simulink model "test"  (Simulink 8.4)
settings: Solver=ode45  StartTime=0.0  StopTime=10.0  RelTol=1e-3
settings Model: Creator=fanwenjun  LastModifiedBy=fanwenjun
settings DataIOCC: SignalLoggingSaveFormat=Dataset
settings OptimizationCC: ExpressionDepthLimit=128
settings DebuggingCC: UnderspecifiedInitializationDetection=Simplified  MergeDetectMultiDrivingBlocksExec=error  FcnCallInpInsideContextMsg=EnableAllAsError  StateNameClashWarn=none
settings GRTTargetCC: CombineOutputUpdateFcns=on  GRTInterface=off

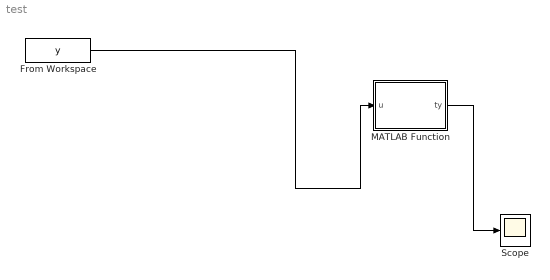
== system test ==
  From Workspace : FromWorkspace  VariableName=y  SampleTime=0
  MATLAB Function : MATLAB Function  TreatAsAtomicUnit=on
  Scope : Scope
  wires:
  From Workspace/1 -> MATLAB Function/1(u)
  MATLAB Function/1(ty) -> Scope/1

== matlab function MATLAB Function ==
  data: u input double; ty output double
function ty = fcn(u)
%#codegen
y=u;
Rpeak=peakDetection(y,512);
for i=1:length(Rpeak)-1
    Tpnot(i)=Rpeak(i)+floor((Rpeak(i+1)-Rpeak(i))/2);
end
dd=cc(Tpnot);
xi=1:1:59001;
wi=interp1(Tpnot,dd,xi,'cubic');
ty=cc-wi;
